simulink model "Cau_3_1617"  (R2016b)
settings: Solver=ode4  StartTime=0.0  StopTime=2  FixedStep=1e-4  RelTol=1e-3
settings Model: Creator=ADMIN  LastModifiedBy=ADMIN

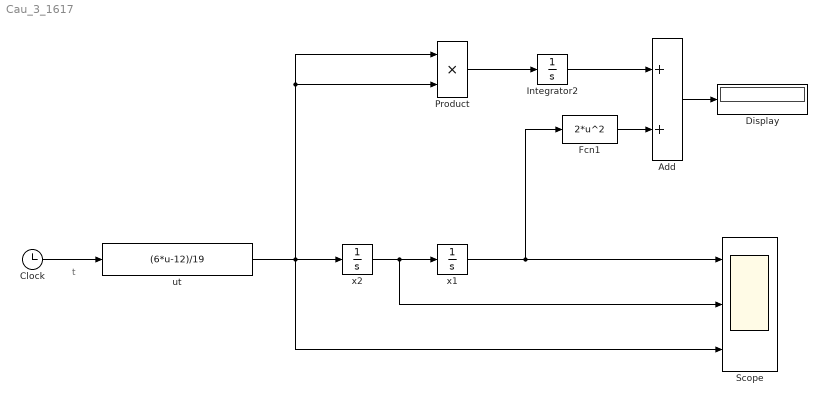
== system Cau_3_1617 ==
  note: t
  Add : Sum
  Clock : Clock
  Display : Display
  Fcn1 : Fcn  Expr=2*u^2
  Integrator2 : Integrator
  Product : Product
  Scope : Scope  NumInputPorts=3
  ut : Fcn  Expr=(6*u-12)/19
  x1 : Integrator  InitialCondition=-1
  x2 : Integrator  InitialCondition=1
  wires:
  Clock/1 -> ut/1
  ut/1 -> Scope/3, Product/2, Product/1, x2/1
  x2/1 -> Scope/2, x1/1
  Add/1 -> Display/1
  Product/1 -> Integrator2/1
  x1/1 -> Fcn1/1, Scope/1
  Fcn1/1 -> Add/2
  Integrator2/1 -> Add/1
